simulink model "observer"  (R2023b)
settings: Solver=VariableStepAuto  StartTime=0.0  StopTime=50.0  RelTol=1e-3
values from neighbouring files (symbols this model uses):
  A = [ -8.8487+(a-b)/5,           -0.0399,                     -5.55+(c+d)/10,               3.5846 ... (first row only)    [Q3.m]    (also in state_observer.m = parameters{1})
  B = [0.0564+b/(10+c),                       0.0319 ... (first row only)    [Q3.m]    (also in state_observer.m = parameters{2})
  C = [-3.2988,              -2.1932+(10*c+d)/(100+5*a),  0.037,      -0.0109 ... (first row only)    [Q3.m]    (also in state_observer.m = parameters{3})
  x0 = parameters{5}    [state_observer.m]
undefined symbols (not defined in the file or in its folder): K_LQR, L_estimator
settings Model: Creator=wyton  LastModifiedBy=shipingguo
settings SolverCC: AlgebraicLoopSolver=TrustRegion
settings OptimizationCC: ReuseModelBlockBuffer=off
settings DebuggingCC: UnconnectedInputMsg=warning  UnconnectedOutputMsg=warning  UnconnectedLineMsg=warning
settings ModelReferenceCC: EnableRefExpFcnMdlSchedulingChecks=on
settings RTWCC: DLArmComputeVersion=19.05

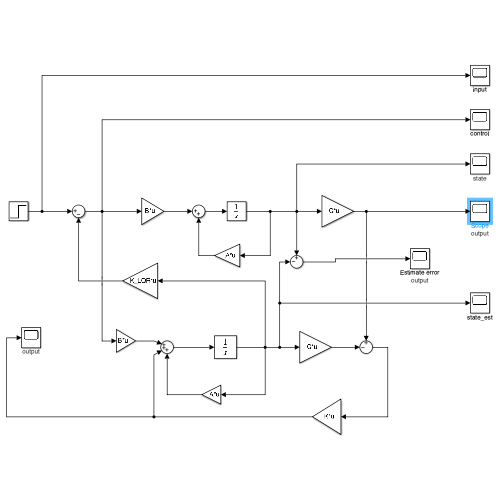
[thumbnail: Simulink's stored preview of the top-level diagram]
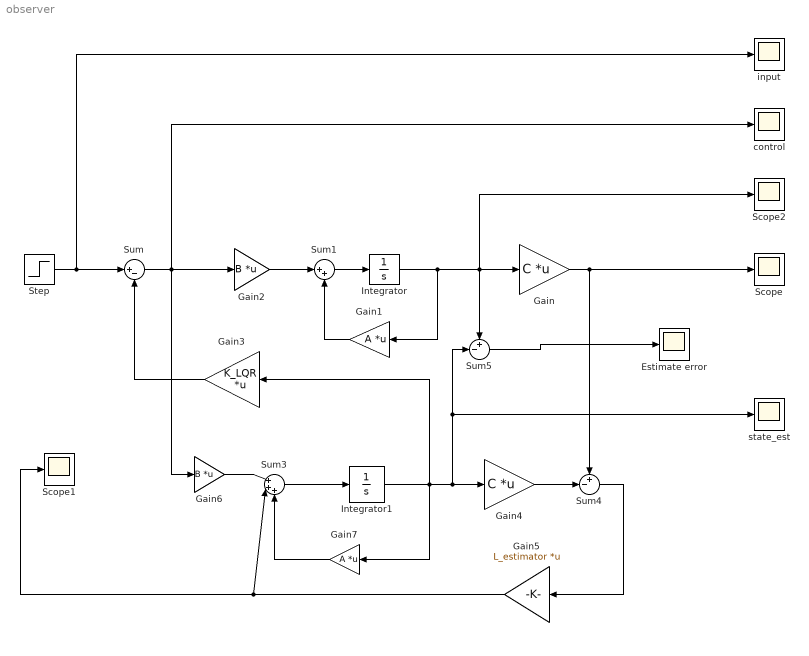
== system observer ==
  Estimate error : Scope
      settings: AttributesFormatString=output
  Gain : Gain  Gain=C  Multiplication=Matrix(K*u)
  Gain1 : Gain  Gain=A  Multiplication=Matrix(K*u)
  Gain2 : Gain  Tag=B  Gain=B  Multiplication=Matrix(K*u)
  Gain3 : Gain  Gain=K_LQR  Multiplication=Matrix(K*u)
  Gain4 : Gain  Gain=C  Multiplication=Matrix(K*u)
  Gain5 : Gain  Gain=L_estimator  Multiplication=Matrix(K*u)
  Gain6 : Gain  Gain=B  Multiplication=Matrix(K*u)
  Gain7 : Gain  Gain=A  Multiplication=Matrix(K*u)
  Integrator : Integrator  InitialCondition=x0
  Integrator1 : Integrator
  Scope : Scope
      settings: AttributesFormatString=output
  Scope1 : Scope
      settings: AttributesFormatString=output
  Scope2 : Scope
      settings: AttributesFormatString=state
  Step : Step  Time=0  Before=[0,0]  After=[1;0]  SampleTime=0
  Sum : Sum  Inputs=|+-
  Sum1 : Sum  Inputs=|++
  Sum3 : Sum  Inputs=|+++
  Sum4 : Sum  Inputs=+-|
  Sum5 : Sum  Inputs=+-|
  control : Scope
  input : Scope
  state_est : Scope
  wires:
  Step/1 -> input/1, Sum/1
  Sum/1 -> control/1, Gain6/1, Gain2/1
  Sum1/1 -> Integrator/1
  Gain2/1 -> Sum1/1
  Gain1/1 -> Sum1/2
  Gain/1 -> Sum4/1, Scope/1
  Gain3/1 -> Sum/2
  Gain6/1 -> Sum3/1
  Gain5/1 -> Scope1/1, Sum3/2
  Gain7/1 -> Sum3/3
  Sum3/1 -> Integrator1/1
  Integrator1/1 -> Gain3/1, state_est/1, Sum5/2, Gain4/1, Gain7/1
  Gain4/1 -> Sum4/2
  Sum5/1 -> Estimate error/1
  Sum4/1 -> Gain5/1
  Integrator/1 -> Sum5/1, Scope2/1, Gain/1, Gain1/1
